simulink model "ClosedLoop_CqCscCi"  (R2023b)
settings: Solver=VariableStepAuto  StartTime=0.0  StopTime=10.0  RelTol=1e-3
libraries: cstblocks x5
settings Model: Creator=randolf  LastModifiedBy=randolf

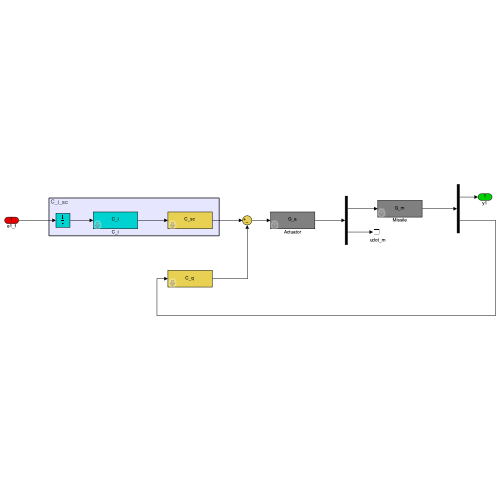
[thumbnail: Simulink's stored preview of the top-level diagram]
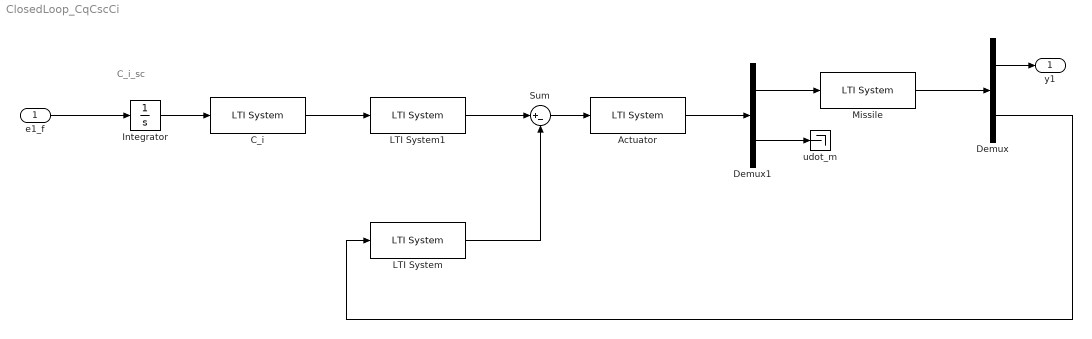
== system ClosedLoop_CqCscCi ==
  note: C_i_sc
  e1_f : Inport
  Actuator : cstblocks/LTI System  sys=G_a  IC=[]  PadeOrder=0
  C_i : cstblocks/LTI System  sys=C_i  IC=[]  PadeOrder=0
  Demux : Demux  Outputs=2
  Demux1 : Demux  Outputs=2
  Integrator : Integrator
  LTI System : cstblocks/LTI System  sys=C_q  IC=[]  PadeOrder=0
  LTI System1 : cstblocks/LTI System  sys=C_sc  IC=[]  PadeOrder=0
  Missile : cstblocks/LTI System  sys=G_m  IC=[]  PadeOrder=0
  Sum : Sum  Inputs=|+-
  udot_m : Terminator
  y1 : Outport
  wires:
  LTI System1/1 -> Sum/1
  Missile/1 -> Demux/1
  Demux/1 -> y1/1
  LTI System/1 -> Sum/2
  Actuator/1 -> Demux1/1
  Sum/1 -> Actuator/1
  Demux1/1 -> Missile/1
  Demux/2 -> LTI System/1
  Demux1/2 -> udot_m/1
  Integrator/1 -> C_i/1
  C_i/1 -> LTI System1/1
  e1_f/1 -> Integrator/1
